simulink model "SW1"  (R2021a)
settings: Solver=ode4  StartTime=0.0  StopTime=40  FixedStep=0.01  RelTol=1e-3
settings Model: Creator=samu  LastModifiedBy=samu

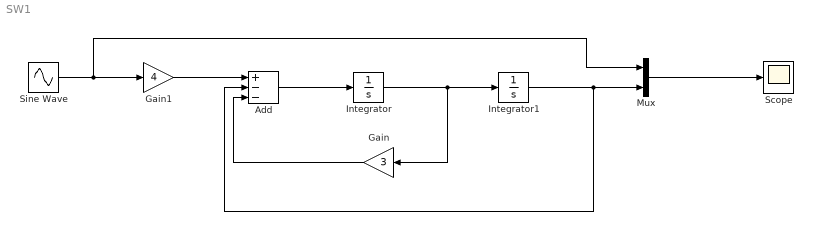
== system SW1 ==
  Add : Sum  Inputs=+--
  Gain : Gain  Gain=3
  Gain1 : Gain  Gain=4
  Integrator : Integrator  InitialCondition=-2
  Integrator1 : Integrator  InitialCondition=4
  Mux : Mux  Inputs=2
  Scope : Scope
  Sine Wave : Sin  SampleTime=0
  wires:
  Integrator/1 -> Gain/1, Integrator1/1
  Gain1/1 -> Add/1
  Mux/1 -> Scope/1
  Sine Wave/1 -> Mux/1, Gain1/1
  Integrator1/1 -> Add/2, Mux/2
  Gain/1 -> Add/3
  Add/1 -> Integrator/1
